simulink model "learnFSM"  (R2017a)
settings: Solver=FixedStepAuto  StartTime=0.0  StopTime=inf  RelTol=1e-3
settings Model: Creator=teobaiguera  LastModifiedBy=teobaiguera

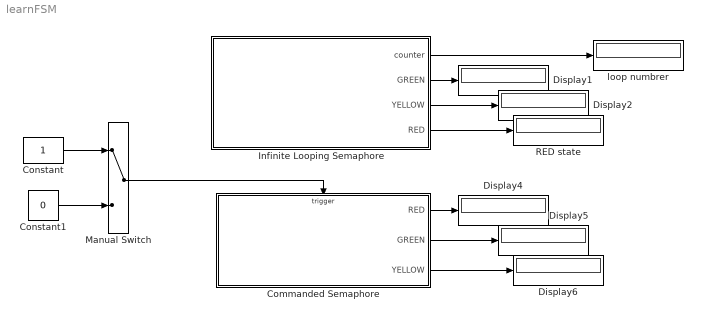
== system learnFSM ==
  Commanded Semaphore : Stateflow chart  TreatAsAtomicUnit=on
  Constant : Constant
  Constant1 : Constant  Value=0
  Display{1..2,4..6} (5 alike) : Display
  Infinite Looping Semaphore : Stateflow chart  TreatAsAtomicUnit=on
  Manual Switch : ManualSwitch
  RED state : Display
  loop numbrer : Display
  wires:
  Constant/1 -> Manual Switch/1
  Constant1/1 -> Manual Switch/2
  Manual Switch/1 -> Commanded Semaphore/Trigger
  Infinite Looping Semaphore/1(counter) -> loop numbrer/1
  Infinite Looping Semaphore/2(" GREEN") -> Display1/1
  Infinite Looping Semaphore/4(" RED") -> RED state/1
  Infinite Looping Semaphore/3(" YELLOW") -> Display2/1
  Commanded Semaphore/1(" RED") -> Display4/1
  Commanded Semaphore/2(" GREEN") -> Display5/1
  Commanded Semaphore/3(" YELLOW") -> Display6/1

== stateflow chart learnFSM/Infinite Looping Semaphore ==
  settings: executeAtInitialization=1
  state GREEN
  state RED
  state YELLOW
  (default) -> RED
  GREEN -> RED : after(1000,sec)
  RED -> YELLOW : after(1000,sec){counter = counter+1}
  YELLOW -> GREEN : after(1000,sec)
  data: counter output =0; GREEN output boolean; YELLOW output boolean; RED output boolean

== stateflow chart learnFSM/Commanded Semaphore ==
  state RED
  state YELLOW
  state GREEN
  YELLOW -> RED : sm_data[after(10,sec)]
  (default) -> RED
  RED -> GREEN : sm_data[after(10,sec)]
  GREEN -> YELLOW : sm_data[after(10,sec)]
  data: counter local double; RED output boolean; GREEN output boolean; YELLOW output boolean
  events: sm_data input EITHER_EDGE_EVENT
